simulink model "Linear_n10295399"  (R2020b)
settings: Solver=ode45  StartTime=0.0  StopTime=40  MaxStep=0.001  RelTol=1e-3  EnableMultiTasking=on
values from neighbouring files (symbols this model uses):
  A = [0 1 0 0 ... (first row only)    [main_n10295399.m]
  B = [0 ... (first row only)    [main_n10295399.m]
  C = [1 0 0 0 ... (first row only)    [main_n10295399.m]
  controller_enabled = 1    [main_n10295399.m]
  Disturbance_enabled = 1    [main_n10295399.m]
  K = place(A,B,p)    [main_n10295399.m]
  L_con = place(A', C', desiredPoles)'    [main_n10295399.m]
  use_state_estimates = 1    [main_n10295399.m]
  x0 = [10*pi/180 0 0.1 0]'    [main_n10295399.m]
  x_bar = [0 0 0 0]'    [main_n10295399.m]
settings Model: Creator=khalil
settings DataIOCC: SaveFormat=Array  ReturnWorkspaceOutputs=off
settings OptimizationCC: LifeSpan=inf
settings DebuggingCC: UnderspecifiedInitializationDetection=Classic  MergeDetectMultiDrivingBlocksExec=none  SolverPrmCheckMsg=warning  SFUnexpectedBacktrackingDiag=warning  SFNoUnconditionalDefaultTransitionDiag=warning  SFExecutionAtInitializationDiag=none  ArithmeticOperatorsInVariantConditions=warning
settings HardwareCC: ProdBitPerPointer=32  ProdBitPerSizeT=32  ProdBitPerPtrDiffT=32  ProdLargestAtomicFloat=None  ProdIntDivRoundTo=Undefined  ProdEndianess=Unspecified  ProdWordSize=32  ProdHWDeviceType=32-bit Generic
settings ModelReferenceCC: PropagateSignalLabelsOutOfModel=off
settings SFSimCC: SimUseLocalCustomCode=off  CustomCodeUndefinedFunction=UseInterfaceOnly
settings RTWCC: RTWUseLocalCustomCode=off
settings CodeAppCC: StateflowObjectComments=on
settings GRTTargetCC: TargetLangStandard=C89/C90 (ANSI)
settings ConfigComp: CovMetricSettings=dw  CovSaveCumulativeToWorkspaceVar=on  CovSaveSingleToWorkspaceVar=on  CovExternalEMLEnable=off

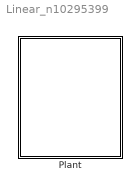
== system Linear_n10295399 ==
  Plant : Subsystem

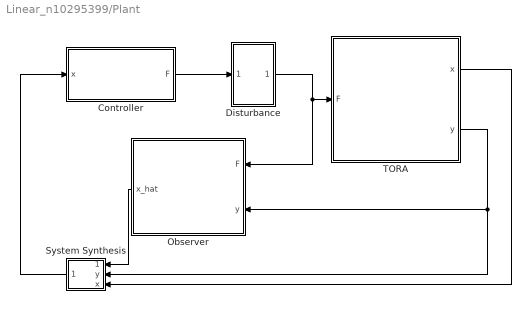
== system Linear_n10295399/Plant ==
  Controller : Subsystem
  Disturbance : Subsystem
  Observer : Subsystem
  System Synthesis : Subsystem
  TORA : Subsystem
      mask Display: image('TORA.png')
  wires:
  TORA/1("x ") -> System Synthesis/3(x)
  Observer/1(x_hat) -> System Synthesis/1(x_hat)
  TORA/2(y) -> System Synthesis/2(y), Observer/2(y)
  System Synthesis/1(x_out) -> Controller/1(x)
  Disturbance/1(Out1) -> Observer/1(F), TORA/1(F)
  Controller/1(F) -> Disturbance/1(In1)

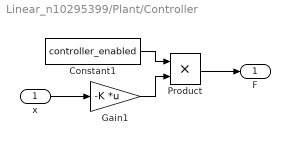
== system Linear_n10295399/Plant/Controller ==
  x : Inport
  Constant1 : Constant  Value=controller_enabled
  Gain1 : Gain  Gain=-K  Multiplication=Matrix(K*u)
  Product : Product
  F : Outport
  wires:
  Gain1/1 -> Product/2
  Product/1 -> F/1
  Constant1/1 -> Product/1
  x/1 -> Gain1/1

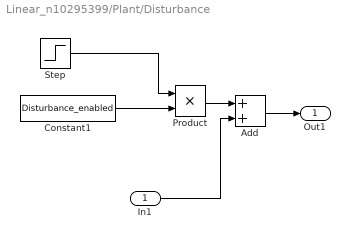
== system Linear_n10295399/Plant/Disturbance ==
  In1 : Inport
  Add : Sum
  Constant1 : Constant  Value=Disturbance_enabled
  Product : Product
  Step : Step  Time=10  After=10  SampleTime=0
  Out1 : Outport
  wires:
  Add/1 -> Out1/1
  Step/1 -> Product/1
  Product/1 -> Add/1
  Constant1/1 -> Product/2
  In1/1 -> Add/2

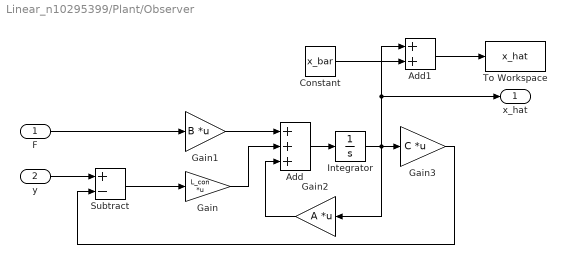
== system Linear_n10295399/Plant/Observer ==
  F : Inport
  y : Inport  Port=2
  Add : Sum  Inputs=+++
  Add1 : Sum
  Constant : Constant  Value=x_bar
  Gain : Gain  Gain=L_con  Multiplication=Matrix(K*u)
  Gain1 : Gain  Gain=B  Multiplication=Matrix(K*u)
  Gain2 : Gain  Gain=A  Multiplication=Matrix(K*u)
  Gain3 : Gain  Gain=C  Multiplication=Matrix(K*u)
  Integrator : Integrator
  Subtract : Sum  Inputs=+-
  To Workspace : ToWorkspace  VariableName=x_hat  SampleTime=-1
  x_hat : Outport  VectorParamsAs1DForOutWhenUnconnected=off
  wires:
  y/1 -> Subtract/1
  Subtract/1 -> Gain/1
  F/1 -> Gain1/1
  Gain1/1 -> Add/1
  Gain/1 -> Add/2
  Add/1 -> Integrator/1
  Gain2/1 -> Add/3
  Gain3/1 -> Subtract/2
  Constant/1 -> Add1/2
  Integrator/1 -> Add1/1, x_hat/1, Gain2/1, Gain3/1
  Add1/1 -> To Workspace/1

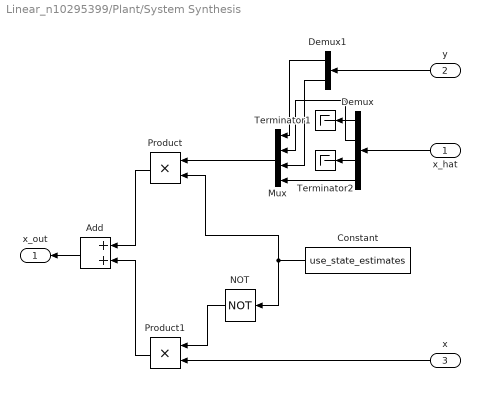
== system Linear_n10295399/Plant/System Synthesis ==
  x_hat : Inport
  y : Inport  Port=2
  x : Inport  Port=3
  Add : Sum
  Constant : Constant  Value=use_state_estimates
  Demux : Demux
  Demux1 : Demux  Outputs=2
  Mux : Mux
  NOT : Logic  Operator=NOT  IconShape=distinctive  AllPortsSameDT=off  OutDataTypeStr=boolean
  Product : Product
  Product1 : Product
  Terminator1 : Terminator
  Terminator2 : Terminator
  x_out : Outport
  wires:
  x_hat/1 -> Demux/1
  Mux/1 -> Product/1
  Constant/1 -> NOT/1, Product/2
  x/1 -> Product1/2
  NOT/1 -> Product1/1
  Add/1 -> x_out/1
  Product/1 -> Add/1
  Product1/1 -> Add/2
  Demux/4 -> Mux/4
  Demux/2 -> Mux/2
  Demux/1 -> Terminator1/1
  Demux/3 -> Terminator2/1
  y/1 -> Demux1/1
  Demux1/1 -> Mux/1
  Demux1/2 -> Mux/3

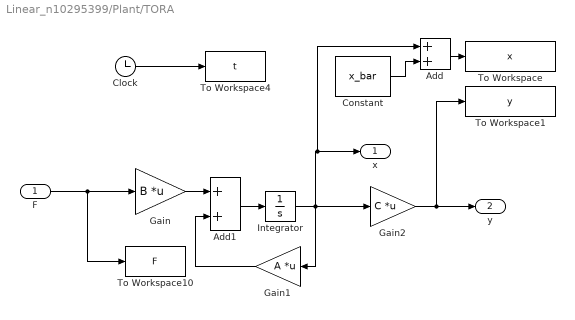
== system Linear_n10295399/Plant/TORA ==
  F : Inport
  Add : Sum
  Add1 : Sum
  Clock : Clock
  Constant : Constant  Value=x_bar
  Gain : Gain  Gain=B  Multiplication=Matrix(K*u)
  Gain1 : Gain  Gain=A  Multiplication=Matrix(K*u)
  Gain2 : Gain  Gain=C  Multiplication=Matrix(K*u)
  Integrator : Integrator  InitialCondition=x0-x_bar
  To Workspace : ToWorkspace  VariableName=x  SampleTime=-1
  To Workspace1 : ToWorkspace  VariableName=y  SampleTime=-1
  To Workspace10 : ToWorkspace  VariableName=F  SampleTime=-1
  To Workspace4 : ToWorkspace  VariableName=t  SampleTime=-1
  "x " : Outport  VectorParamsAs1DForOutWhenUnconnected=off
  y : Outport  Port=2  VectorParamsAs1DForOutWhenUnconnected=off
  wires:
  Constant/1 -> Add/2
  Gain2/1 -> To Workspace1/1, y/1
  Gain/1 -> Add1/1
  Add/1 -> To Workspace/1
  Gain1/1 -> Add1/2
  Add1/1 -> Integrator/1
  Integrator/1 -> Add/1, "x "/1, Gain2/1, Gain1/1
  F/1 -> To Workspace10/1, Gain/1
  Clock/1 -> To Workspace4/1
